simulink model "clik_inverse"  (R2022b)
settings: Solver=ode1  StartTime=0.0  StopTime=4  FixedStep=0.001  RelTol=1e-3
undefined symbols (not defined in the file or in its folder): DiscIntNeverNeededParam, q0, Tc
settings Model: Creator=Xp  LastModifiedBy=anujs
settings SolverCC: AlgebraicLoopSolver=TrustRegion
settings DataIOCC: LimitDataPoints=on  SaveFormat=Array  SignalLoggingSaveFormat=ModelDataLogs  ReturnWorkspaceOutputs=off
settings OptimizationCC: ExpressionDepthLimit=2147483647  InitFltsAndDblsToZero=on  LifeSpan=inf
settings DebuggingCC: SaveWithParameterizedLinksMsg=none  UnderspecifiedInitializationDetection=Classic  MergeDetectMultiDrivingBlocksExec=none  SolverPrmCheckMsg=warning  MultiTaskDSMMsg=warning  MultiTaskCondExecSysMsg=none  FcnCallInpInsideContextMsg=warning  UnconnectedInputMsg=warning  UnconnectedOutputMsg=warning  UnconnectedLineMsg=warning  StateNameClashWarn=warning  SFUnexpectedBacktrackingDiag=warning  SFNoUnconditionalDefaultTransitionDiag=warning  SFExecutionAtInitializationDiag=none  SFMachineParentedDataDiag=warning  ArithmeticOperatorsInVariantConditions=warning
settings HardwareCC: ProdBitPerPointer=32  ProdBitPerSizeT=32  ProdBitPerPtrDiffT=32  ProdLargestAtomicFloat=None  ProdIntDivRoundTo=Undefined  ProdEndianess=Unspecified  ProdWordSize=32  ProdHWDeviceType=32-bit Generic
settings ModelReferenceCC: EnableRefExpFcnMdlSchedulingChecks=on  PropagateSignalLabelsOutOfModel=off
settings SFSimCC: CustomCodeUndefinedFunction=UseInterfaceOnly
settings RTWCC: DLArmComputeVersion=19.05
settings CodeAppCC: StateflowObjectComments=on
settings GRTTargetCC: TargetLangStandard=C89/C90 (ANSI)  CombineOutputUpdateFcns=off  GRTInterface=on
settings ConfigComp: CovMetricSettings=dw  CovSaveCumulativeToWorkspaceVar=on  CovSaveSingleToWorkspaceVar=on

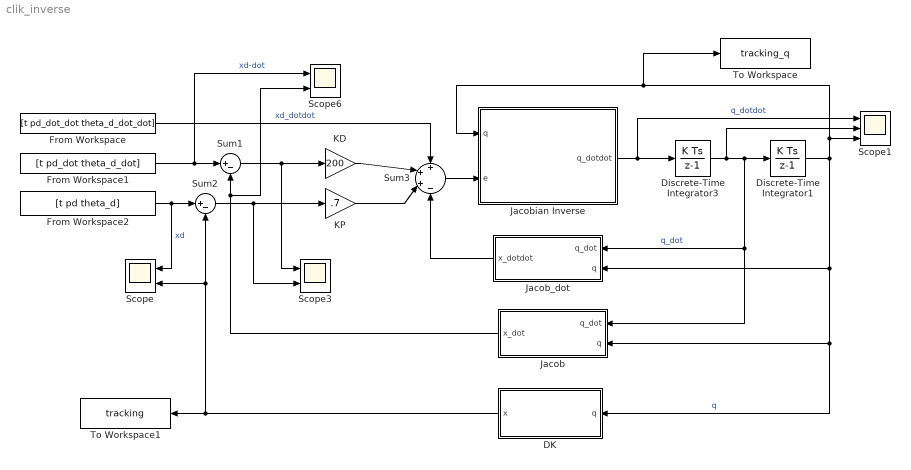
== system clik_inverse ==
  DK : MATLAB Function  TreatAsAtomicUnit=on
  Discrete-Time Integrator1 : DiscreteIntegrator  InitialCondition=q0  SampleTime=Tc  LimitOutput=on  UpperSaturationLimit=[pi/2 pi/4 1 2*pi]'  LowerSaturationLimit=[-pi/2 -pi/2 0.25 -2*pi]'  ICPrevOutput=DiscIntNeverNeededParam  ICPrevScaledInput=DiscIntNeverNeededParam
  Discrete-Time Integrator3 : DiscreteIntegrator  InitialCondition=q0  SampleTime=Tc  LimitOutput=on  UpperSaturationLimit=[pi 3*pi/4 0.75 4*pi]'  LowerSaturationLimit=[-pi -3*pi/4 -0.75 -4*pi]'  ICPrevOutput=DiscIntNeverNeededParam  ICPrevScaledInput=DiscIntNeverNeededParam
  From Workspace : FromWorkspace  VariableName=[t pd_dot_dot theta_d_dot_dot]  SampleTime=Tc  OutputAfterFinalValue=Holding final value
  From Workspace1 : FromWorkspace  VariableName=[t pd_dot theta_d_dot]  SampleTime=Tc  OutputAfterFinalValue=Holding final value
  From Workspace2 : FromWorkspace  VariableName=[t pd theta_d]  SampleTime=Tc  OutputAfterFinalValue=Holding final value
  Jacob : MATLAB Function  TreatAsAtomicUnit=on
  Jacob_dot : MATLAB Function  TreatAsAtomicUnit=on
  Jacobian Inverse : MATLAB Function  TreatAsAtomicUnit=on
  KD : Gain  Gain=200
  KP : Gain  Gain=.7
  Scope : Scope  NumInputPorts=2
  Scope1 : Scope  NumInputPorts=3
  Scope3 : Scope  NumInputPorts=2
  Scope6 : Scope  NumInputPorts=2
  Sum1 : Sum  Inputs=|+-
  Sum2 : Sum  Inputs=|+-
  Sum3 : Sum  Inputs=+++-
  To Workspace : ToWorkspace  VariableName=tracking_q  SampleTime=Tc
  To Workspace1 : ToWorkspace  VariableName=tracking  SampleTime=Tc
  wires:
  Sum1/1 -> Scope3/1, KD/1
  Sum3/1 -> Jacobian Inverse/2(e)
  DK/1(x) -> Sum2/2, Scope/2, To Workspace1/1
  Discrete-Time Integrator1/1 -> Scope1/3, To Workspace/1, Jacobian Inverse/1(q), DK/1(q), Jacob/2(q), Jacob_dot/2(q)  "q"
  KD/1 -> Sum3/2
  Discrete-Time Integrator3/1 -> Scope1/2, Discrete-Time Integrator1/1, Jacob/1(q_dot), Jacob_dot/1(q_dot)  "q_dot"
  Sum2/1 -> KP/1, Scope3/2
  Jacob/1(x_dot) -> Scope6/2, Sum1/2
  KP/1 -> Sum3/3
  From Workspace1/1 -> Scope6/1, Sum1/1  "xd-dot"
  From Workspace2/1 -> Scope/1, Sum2/1  "xd"
  Jacobian Inverse/1(q_dotdot) -> Scope1/1, Discrete-Time Integrator3/1  "q_dotdot"
  From Workspace/1 -> Sum3/1  "xd_dotdot"
  Jacob_dot/1(x_dotdot) -> Sum3/4

== matlab function clik_inverse/Jacobian Inverse ==
  data: q input; e input; q_dotdot output
function q_dotdot = Jacobian_Inverse(q, e)

q_dotdot = jacobian_inverse(q, e);
end

== matlab function clik_inverse/DK ==
  data: q input; x output
function x = Direct_Kinematics(q)

x = direct_kin(q);

== matlab function clik_inverse/Jacob_dot ==
  data: q_dot input; x_dotdot output; q input
function x_dotdot = J_dot(q_dot, q)


x_dotdot = jacobian_dot(q_dot, q);
end

== matlab function clik_inverse/Jacob ==
  data: q_dot input; x_dot output; q input
function x_dot = Jacob(q_dot, q)

%Link length
a1 = 0.5;
a2 = 0.5;

%Joint Variables
t1 = q(1);
t2 = q(2);
d3 = q(3);
t4 = q(4);


Ab0 = [1 0 0 0;0 1 0 0;0 0 1 1;0 0 0 1];
A01 = [cos(t1) -sin(t1) 0 a1*cos(t1); sin(t1) cos(t1) 0 a1*sin(t1); 0 0 1 0; 0 0 0 1];
A12 = [cos(t2) -sin(t2) 0 a2*cos(t2); sin(t2) cos(t2) 0 a2*sin(t2);0 0 1 0;0 0 0 1];
A23 = [1 0 0 0;0 1 0 0;0 0 1 -d3;0 0 0 1];
A34 = [cos(t4) -sin(t4) 0 0;sin(t4) cos(t4) 0 0;0 0 1 0;0 0 0 1];

Ab1 = Ab0*A01;
Ab2 = Ab1*A12;
Ab3 = Ab2*A23;
Ab4 = Ab3*A34;

z0 = [0 0 1]';
z1 = [0 0 1]';
z2 = [0 0 1]';
z3 = [0 0 1]';
z4 = [0 0 1]';

J_1 = cross(z0,Ab4(1:3,4));
J_2 = cross(z1,(Ab4(1:3,4) - Ab1(1:3,4)));
J_4 = cross(z3,(Ab4(1:3,4) - Ab3(1:3,4)));



jac = [[J_1 J_2 z2 J_4];[z0 z1 [0 0 0]' z3]];
Jacobian = ([jac(1:3,:); jac(end,:)]);


x_dot = (Jacobian*q_dot);
